simulink model "Bi_directional_full_bridge_DC_DC_converter"  (R2014a)
settings: Solver=ode45  StartTime=0.0  StopTime=0.1  MaxStep=1e-4  RelTol=1e-3
libraries: powerlib x17, dspstat3 x1
settings Model: CovSFcnEnable=on  Creator=user  LastModifiedBy=范翔宇
settings DataIOCC: LimitDataPoints=off  SaveFormat=StructureWithTime
settings DebuggingCC: MergeDetectMultiDrivingBlocksExec=error  SolverPrmCheckMsg=none  FrameProcessingCompatibilityMsg=error
settings HardwareCC: ProdBitPerPointer=64  ProdLargestAtomicFloat=Float  ProdIntDivRoundTo=Zero  ProdEndianess=LittleEndian  ProdHWDeviceType=Specified
settings ModelReferenceCC: PropagateSignalLabelsOutOfModel=on
settings SimscapeCC: SimscapeNormalizeSystem=off
settings ConfigurationSet: Description=Simscape Multibody

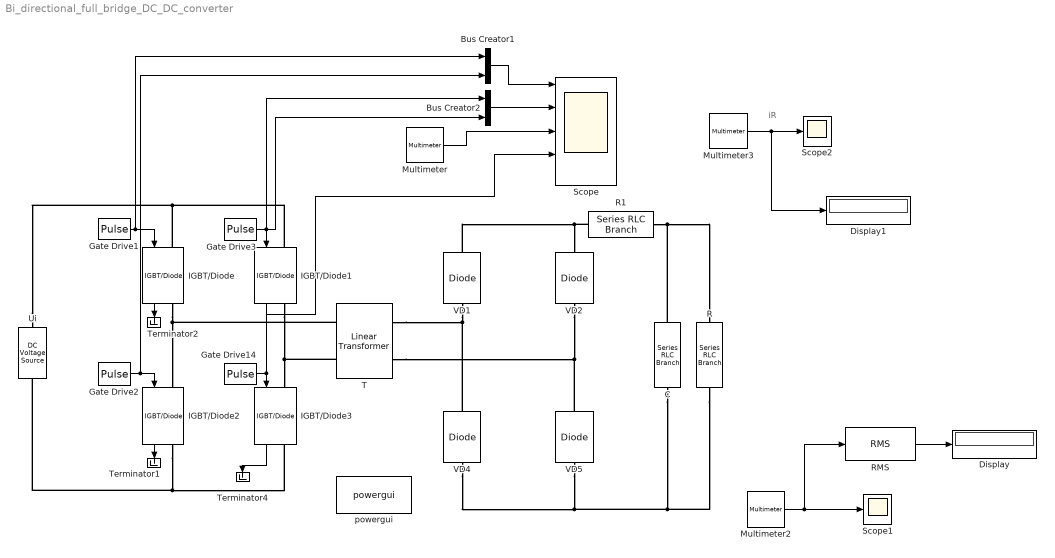
== system Bi_directional_full_bridge_DC_DC_converter ==
  note: iR
  Bus Creator1 : BusCreator  DialogController=Simulink.DDGSource_Bus  Inputs=2
  Bus Creator2 : BusCreator  DialogController=Simulink.DDGSource_Bus  Inputs=2
  C : powerlib/Elements/Series RLC Branch  LConnTagsString=__new0  RConnTagsString=__new0  BranchType=C  Resistance=0  Inductance=0  SetiL0=off  InitialCurrent=0  Capacitance=3e-4  Setx0=off  InitialVoltage=0  Measurements=None
  Display : Display
  Display1 : Display
  Gate Drive1 : DiscretePulseGenerator  PulseType=Time based  Period=5e-5  PulseWidth=25
  Gate Drive14 : DiscretePulseGenerator  PulseType=Time based  Period=5e-5  PulseWidth=25
  Gate Drive2 : DiscretePulseGenerator  PulseType=Time based  Period=5e-5  PulseWidth=25  PhaseDelay=180/7200000
  Gate Drive3 : DiscretePulseGenerator  PulseType=Time based  Period=5e-5  PulseWidth=25  PhaseDelay=180/7200000
  IGBT/Diode{,1..3} (4 alike) : powerlib/Power Electronics/IGBT//Diode  Ron=1e-3  Rs=1e5  Cs=inf  Measurements=on
  Multimeter : powerlib/Measurements/Multimeter  PhasorSimulation=off  OutputType=Complex  sel=[3 7]  L=11  Gain=[1 1]  yselected={'Uw1: T','Iw1: T'};  PSBOutputType=1  PSBequivalent=0  AxesSetting=[0,0.1,-100,100]  Display=0  SavedBlockNames=-11
  Multimeter2 : powerlib/Measurements/Multimeter  PhasorSimulation=off  OutputType=Complex  sel=1  L=11  Gain=1  yselected={'Ub: R'};  PSBOutputType=1  PSBequivalent=0  AxesSetting=[0,0.1,-100,100]  Display=0  SavedBlockNames=-11
  Multimeter3 : powerlib/Measurements/Multimeter  PhasorSimulation=off  OutputType=Complex  sel=5  L=11  Gain=1  yselected={'Ib: R'};  PSBOutputType=1  PSBequivalent=0  AxesSetting=[0,0.1,-100,100]  Display=0  SavedBlockNames=-11
  R : powerlib/Elements/Series RLC Branch  LConnTagsString=__new0  RConnTagsString=__new0  BranchType=R  Resistance=220/30  Inductance=0  SetiL0=off  InitialCurrent=0  Capacitance=inf  Setx0=off  InitialVoltage=0  Measurements=Branch voltage and current
  R1 : powerlib/Elements/Series RLC Branch  LConnTagsString=__new0  RConnTagsString=__new0  BranchType=L  Resistance=220/30  Inductance=1e-7  SetiL0=off  InitialCurrent=0  Capacitance=inf  Setx0=off  InitialVoltage=0  Measurements=Branch voltage and current
  RMS : dspstat3/RMS  run=off  directionMode=Each column  dimension=1  InputProcessing=Columns as channels (frame based)  reset_popup=None  treatSBRowAsCol=off
  Scope : Scope  NumInputPorts=5
      settings: TimeRange=0.0001  MaxDataPoints=5000  SaveToWorkspace=off  YMin=-0.125~-0.125~-0.37494~-1.83735~-1.00000  YMax=1.125~1.125~0.37494~13.53782~1.00000  SampleTime=-1
  Scope1 : Scope
      settings: TimeRange=auto  MaxDataPoints=5000  SaveToWorkspace=off  SaveName=ScopeData2  YMin=-25.77848  YMax=232.00629  SampleTime=-1  Grid=off
  Scope2 : Scope
      settings: TimeRange=auto  MaxDataPoints=5000  SaveToWorkspace=off  YMin=27.94273  YMax=28.14189  SampleTime=-1  Grid=off
  T : powerlib/Elements/Linear Transformer  UNITS=pu  NominalPower=[500 20000 ]  winding1=[200 0 0]  winding2=[4900 0 0]  ThreeWindings=off  winding3=[11000 0 0]  RmLm=[1e6 1e6]  Measurements=All voltages and currents  DataType=off
  Terminator1 : Terminator
  Terminator2 : Terminator
  Terminator4 : Terminator
  Ui : powerlib/Electrical Sources/DC Voltage Source  Amplitude=12  Measurements=None
  VD{1..2,4..5} (4 alike) : powerlib/Power Electronics/Diode  Ron=0.001  Lon=0  Vf=0  IC=0  UseSnubber=off  Rs=500  Cs=1e-9  Measurements=off
  powergui : powerlib/powergui  Priority=1  SimulationMode=Continuous  SampleTime=50e-6  frequency=60  Iterations=50  frequencyindice=0  Pbase=100e6  ErrMax=1e-4  UnitsV=kV  UnitsW=MW  buscounter=0  FunctionMessages=off  echomessages=off  EnableUseOfTLC=off  CurrentSourceSwitches=off  DisableSnubberDevices=off  DisableRonSwitches=off  DisableVfSwitches=off  DisplayEquations=off  SolverType=Tustin/Backward Euler (TBE)  Interpol=off  ExternalGateDelay=off  methode=off  Ts=100  x0status=blocks  SPID=on  SwTol=0  HookPort=off  RestoreLinks=warning  ResistiveCurrentMeasurement=off  Frange=[0:2:500]  Ylog=off  Xlog=on  ShowGrid=off  save=off  variable=ZData  structure=0  ZoomFFT=off  StartTime=0.0  cycles=1  DisplayStyle=1  fundamental=60  FreqAxis=off  MaxFrequency=1000  frequencyindicesteady=1  RmsSteady=1  display=off
  wires:
  Gate Drive1/1 -> IGBT/Diode/1, Bus Creator1/1
  Multimeter/1 -> Scope/3
  Gate Drive2/1 -> IGBT/Diode2/1, Bus Creator1/2
  IGBT/Diode2/1 -> Terminator1/1
  IGBT/Diode3/1 -> Terminator4/1
  Gate Drive3/1 -> Bus Creator2/2, IGBT/Diode1/1
  Gate Drive14/1 -> Bus Creator2/1, IGBT/Diode3/1
  Bus Creator1/1 -> Scope/1
  Bus Creator2/1 -> Scope/2
  IGBT/Diode1/1 -> Scope/4
  Multimeter2/1 -> RMS/1, Scope1/1
  Multimeter3/1 -> Scope2/1, Display1/1
  IGBT/Diode/1 -> Terminator2/1
  RMS/1 -> Display/1
  connections:
  Ui/LConn1 -- IGBT/Diode3/RConn1 -- IGBT/Diode2/RConn1
  IGBT/Diode1/RConn1 -- T/LConn2 -- IGBT/Diode3/LConn1
  IGBT/Diode/RConn1 -- T/LConn1 -- IGBT/Diode2/LConn1
  Ui/RConn1 -- IGBT/Diode1/LConn1 -- IGBT/Diode/LConn1
  C/RConn1 -- R/RConn1 -- VD5/LConn1 -- VD4/LConn1
  T/RConn2 -- VD5/RConn1 -- VD2/LConn1
  T/RConn1 -- VD4/RConn1 -- VD1/LConn1
  VD1/RConn1 -- VD2/RConn1 -- R1/RConn1
  C/LConn1 -- R1/LConn1 -- R/LConn1
